simulink model "coupled_tanks"  (R2015b)
settings: Solver=VariableStepAuto  StartTime=0.0  StopTime=300  FixedStep=0.1  RelTol=1e-3
settings Model: ExtModeTrigMode=oneshot  ExtModeArmWhenConnect=off  Creator=magudelo  LastModifiedBy=Mauricio
settings DataIOCC: LimitDataPoints=off  SaveFormat=Array  SignalLoggingSaveFormat=ModelDataLogs
settings OptimizationCC: BlockReduction=off  BooleanDataType=off  ExpressionDepthLimit=2147483647
settings DebuggingCC: SaveWithParameterizedLinksMsg=none  UnderspecifiedInitializationDetection=Classic  MergeDetectMultiDrivingBlocksExec=none  SignalResolutionControl=TryResolveAllWithWarning  MultiTaskDSMMsg=warning  MultiTaskCondExecSysMsg=none  FcnCallInpInsideContextMsg=UseLocalSettings  StateNameClashWarn=warning
settings HardwareCC: ProdBitPerPointer=32  ProdLargestAtomicFloat=None  ProdIntDivRoundTo=Undefined  ProdEndianess=Unspecified  ProdWordSize=32  ProdHWDeviceType=32-bit Generic  TargetUnknown=on
settings GRTTargetCC: GeneratePreprocessorConditionals=Disable all  CombineOutputUpdateFcns=off  GRTInterface=on
settings ConfigComp: CovModelRefEnable=Off

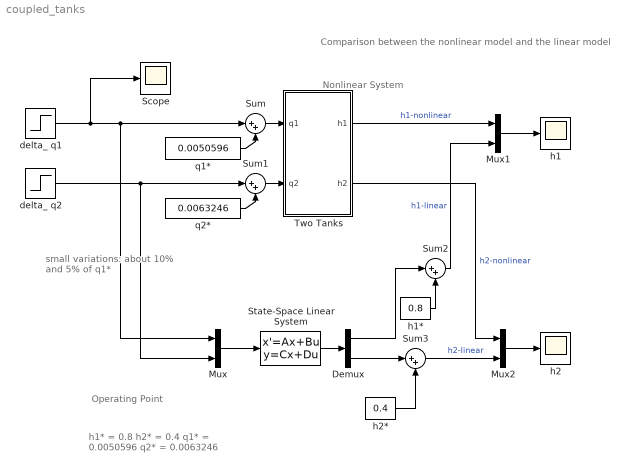
== system coupled_tanks ==
  note: Nonlinear System
  note: Comparison between the nonlinear model and the linear model
  note: Operating Point
  note: h1* = 0.8
      | h2* =  0.4
      | q1* = 0.0050596
      | q2* = 0.0063246
  note: small variations: about
      | 10% and 5% of q1*
  Demux : Demux  Outputs=2
  Mux : Mux  Inputs=2
  Mux1 : Mux  Inputs=2
  Mux2 : Mux  Inputs=2
  Scope : Scope
  State-Space Linear System : StateSpace  A=[-0.0891 0.0891; 0.0891 -0.2895]  B=[14.0845 0; 0 14.0845]  C=eye(2,2)  D=zeros(2,2)  X0=0
  Sum{,1..3} (4 alike) : Sum  Inputs=|++  SaturateOnIntegerOverflow=on  InputSameDT=on  OutDataTypeStr=Inherit: Same as first input
  Two Tanks : Subsystem  mask(Tanks systems){A1=0.071, A2=0.071, k1=0.008, k2=0.018, h10=0.8, h20=0.4}
      mask prompts: A1 "Cross sectional area of Tank 1 :"; A2 "Cross sectional area of Tank 2  :"; k1 "Valve coefficient k1 :"; k2 "Valve coeficient k2 :"; h10 "Initial level for Tank 1:"; h20 "Initial level for Tank 2 :"
      mask help:
      | Sistema de 2 tanques acoplados.
      |
      | Oscar Mauricio Agudelo Mañozca
      | OMAM/2002
  delta_ q1 : Step  Time=150  Before=0.0005*(1)  After=0.00025*(1)  SampleTime=0
  delta_ q2 : Step  Time=150  Before=0.0005*(1)  After=0.00025*(1)  SampleTime=0
  h1 : Scope
  h1* : Constant  Value=0.8
  h2 : Scope
  h2* : Constant  Value=0.4
  q1* : Constant  Value=0.0050596
  q2* : Constant  Value=0.0063246
  wires:
  Sum/1 -> Two Tanks/1(q1)
  q1*/1 -> Sum/2
  Sum1/1 -> Two Tanks/2(q2)
  q2*/1 -> Sum1/2
  delta_ q1/1 -> Sum/1, Mux/1, Scope/1
  delta_ q2/1 -> Sum1/1, Mux/2
  Mux1/1 -> h1/1
  Two Tanks/1(h1) -> Mux1/1  "h1-nonlinear"
  State-Space Linear System/1 -> Demux/1
  Demux/2 -> Sum3/1
  h2*/1 -> Sum3/2
  Sum3/1 -> Mux2/2  "h2-linear"
  Two Tanks/2(h2) -> Mux2/1  "h2-nonlinear"
  Mux2/1 -> h2/1
  Mux/1 -> State-Space Linear System/1
  h1*/1 -> Sum2/2
  Demux/1 -> Sum2/1
  Sum2/1 -> Mux1/2  "h1-linear"

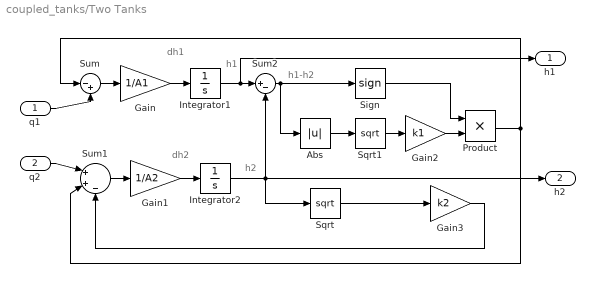
== system coupled_tanks/Two Tanks ==
  note: h1-h2
  note: h2
  note: dh2
  note: h1
  note: dh1
  q1 : Inport
  q2 : Inport  Port=2
  Abs : Abs  SaturateOnIntegerOverflow=on
  Gain : Gain  Gain=1/A1  SaturateOnIntegerOverflow=on  OutDataTypeStr=Inherit: Same as input  ParamDataTypeStr=Inherit: Same as input
  Gain1 : Gain  Gain=1/A2  SaturateOnIntegerOverflow=on  OutDataTypeStr=Inherit: Same as input  ParamDataTypeStr=Inherit: Same as input
  Gain2 : Gain  Gain=k1  SaturateOnIntegerOverflow=on  OutDataTypeStr=Inherit: Same as input  ParamDataTypeStr=Inherit: Same as input
  Gain3 : Gain  Gain=k2  SaturateOnIntegerOverflow=on  OutDataTypeStr=Inherit: Same as input  ParamDataTypeStr=Inherit: Same as input
  Integrator1 : Integrator  InitialCondition=h10  LimitOutput=on  LowerSaturationLimit=0
  Integrator2 : Integrator  InitialCondition=h20  LimitOutput=on  LowerSaturationLimit=0
  Product : Product  SaturateOnIntegerOverflow=on  RndMeth=Zero  InputSameDT=on  OutDataTypeStr=Inherit: Same as first input
  Sign : Signum
  Sqrt : Sqrt  SaturateOnIntegerOverflow=on
  Sqrt1 : Sqrt  SaturateOnIntegerOverflow=on
  Sum : Sum  Inputs=|-+  SaturateOnIntegerOverflow=on  InputSameDT=on  OutDataTypeStr=Inherit: Same as first input
  Sum1 : Sum  Inputs=|++-  SaturateOnIntegerOverflow=on  InputSameDT=on  OutDataTypeStr=Inherit: Same as first input
  Sum2 : Sum  Inputs=|+-  SaturateOnIntegerOverflow=on  InputSameDT=on  OutDataTypeStr=Inherit: Same as first input
  h1 : Outport
  h2 : Outport  Port=2
  wires:
  Sum/1 -> Gain/1
  Gain/1 -> Integrator1/1
  Product/1 -> Sum/1, Sum1/2
  Integrator1/1 -> Sum2/1, h1/1
  q1/1 -> Sum/2
  Sum2/1 -> Abs/1, Sign/1
  Abs/1 -> Sqrt1/1
  Sqrt1/1 -> Gain2/1
  Gain2/1 -> Product/2
  Sign/1 -> Product/1
  Sum1/1 -> Gain1/1
  Gain1/1 -> Integrator2/1
  q2/1 -> Sum1/1
  Gain3/1 -> Sum1/3
  Integrator2/1 -> Sqrt/1, Sum2/2, h2/1
  Sqrt/1 -> Gain3/1
